simulink model "ASS_Final"  (R2019a)
settings: Solver=VariableStepAuto  StartTime=0.0  StopTime=30  RelTol=1e-3
values from neighbouring files (symbols this model uses):
  B1 = 100    [ASS_Final_parametros.m]
  B2 = 2000    [ASS_Final_parametros.m]
  eta = 0.92    [ASS_Final_parametros.m]
  io = 0    [ASS_Final_parametros.m]
  J = 0.15e-6    (= 1.5e-07)    [ASS_Final_parametros.m]
  k = 0.456    [ASS_Final_parametros.m]
  K1 = 125000    [ASS_Final_parametros.m]
  K2 = 28000    [ASS_Final_parametros.m]
  L = 20e-3    (= 0.02)    [ASS_Final_parametros.m]
  M1 = 40    [ASS_Final_parametros.m]
  M2 = 250    [ASS_Final_parametros.m]
  r = 0.4    [ASS_Final_parametros.m]
settings Model: Creator=luiso  LastModifiedBy=Amilcar A

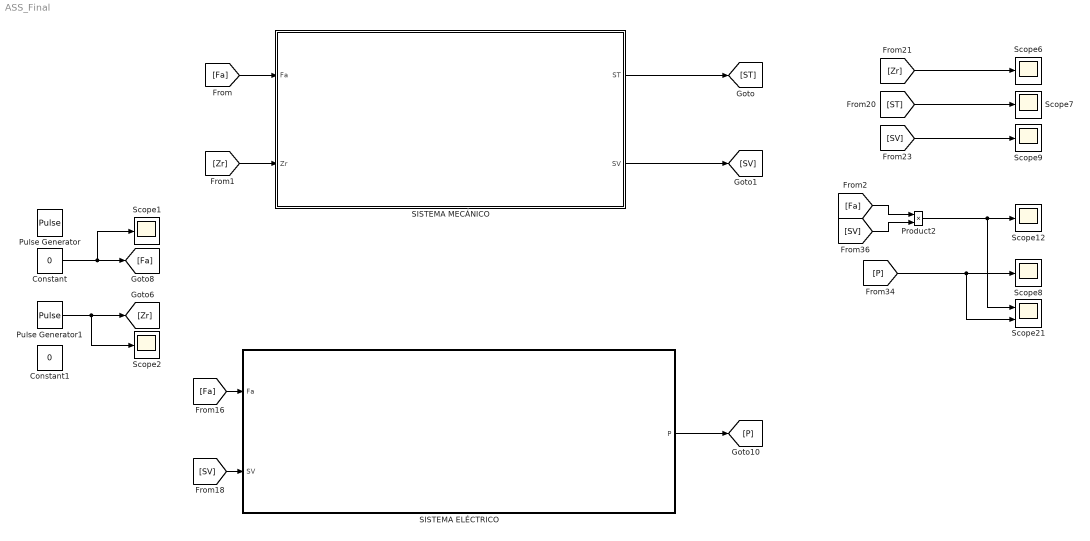
== system ASS_Final ==
  Constant : Constant  Value=0
  Constant1 : Constant  Value=0
  Product2 : Product
  Pulse Generator : DiscretePulseGenerator  PulseType=Time based  Amplitude=10  Period=10  PulseWidth=50
  Pulse Generator1 : DiscretePulseGenerator  PulseType=Time based  Amplitude=10e-4  Period=10  PulseWidth=50
  SISTEMA ELÉCTRICO : Subsystem
  SISTEMA MECÁNICO : Subsystem
  Scope{1..2,6..9,12} (7 alike) : Scope
  Scope21 : Scope  NumInputPorts=2
  wires:
  Pulse Generator1/1 -> Scope2/1, [Zr]
  Constant/1 -> Scope1/1, [Fa]
  [SV] -> Product2/2
  Product2/1 -> Scope21/1, Scope12/1
  [P] -> Scope21/2, Scope8/1
  [ST] -> Scope7/1
  [Zr] -> Scope6/1
  [SV] -> Scope9/1
  [Fa] -> SISTEMA MECÁNICO/1(Fa)
  [Zr] -> SISTEMA MECÁNICO/2(Zr)
  SISTEMA MECÁNICO/1(ST) -> [ST]
  SISTEMA MECÁNICO/2(SV) -> [SV]
  [Fa] -> SISTEMA ELÉCTRICO/1(Fa)
  [SV] -> SISTEMA ELÉCTRICO/2(SV)
  SISTEMA ELÉCTRICO/1(P) -> [P]
  [Fa] -> Product2/1

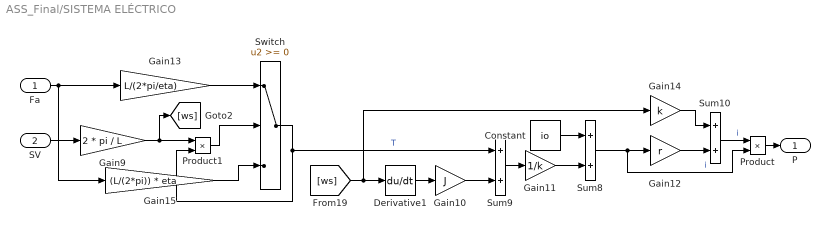
== system ASS_Final/SISTEMA ELÉCTRICO ==
  Fa : Inport
  SV : Inport  Port=2
  Constant : Constant  Value=io
  Derivative1 : Derivative
  Gain10 : Gain  Gain=J
  Gain11 : Gain  Gain=1/k
  Gain12 : Gain  Gain=r
  Gain13 : Gain  Gain=L/(2*pi/eta)
  Gain14 : Gain  Gain=k
  Gain15 : Gain  Gain=(L/(2*pi)) * eta
  Gain9 : Gain  Gain=2 * pi / L
  Product : Product
  Product1 : Product
  Sum10 : Sum
  Sum8 : Sum
  Sum9 : Sum
  Switch : Switch
  P : Outport
  wires:
  Constant/1 -> Sum8/1
  [ws] -> Gain14/1, Derivative1/1
  Gain15/1 -> Switch/3
  Switch/1 -> Product1/2, Sum9/1  "T"
  Gain12/1 -> Sum10/2
  Fa/1 -> Gain15/1, Gain13/1
  Sum9/1 -> Gain11/1
  Derivative1/1 -> Gain10/1
  Sum10/1 -> Product/1  "i"
  Gain10/1 -> Sum9/2
  Gain11/1 -> Sum8/2
  Product1/1 -> Switch/2
  Gain13/1 -> Switch/1
  Gain14/1 -> Sum10/1
  Product/1 -> P/1
  Sum8/1 -> Product/2, Gain12/1  "i"
  Gain9/1 -> [ws], Product1/1
  SV/1 -> Gain9/1

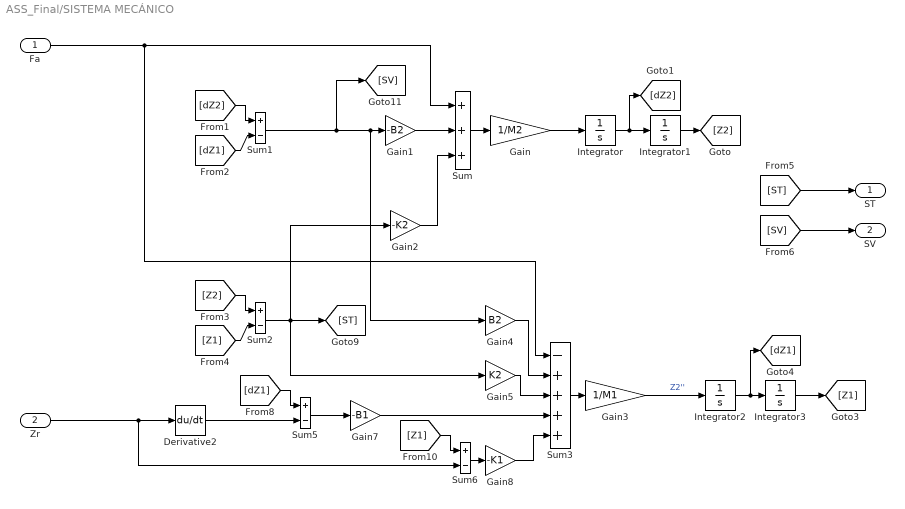
== system ASS_Final/SISTEMA MECÁNICO ==
  Fa : Inport
  Zr : Inport  Port=2
  Derivative2 : Derivative
  Gain : Gain  Gain=1/M2
  Gain1 : Gain  Gain=-B2
  Gain2 : Gain  Gain=-K2
  Gain3 : Gain  Gain=1/M1
  Gain4 : Gain  Gain=B2
  Gain5 : Gain  Gain=K2
  Gain7 : Gain  Gain=-B1
  Gain8 : Gain  Gain=-K1
  Integrator{,1..3} (4 alike) : Integrator
  Sum : Sum  Inputs=+++
  Sum{1..2,5..6} (4 alike) : Sum  Inputs=+-
  Sum3 : Sum  Inputs=-++++
  ST : Outport
  SV : Outport  Port=2
  wires:
  Gain/1 -> Integrator/1
  Sum1/1 -> Gain1/1, Gain4/1, [SV]
  Gain7/1 -> Sum3/4
  Sum2/1 -> Gain2/1, [ST], Gain5/1
  Gain8/1 -> Sum3/5
  Integrator3/1 -> [Z1]
  Sum6/1 -> Gain8/1
  Derivative2/1 -> Sum5/2
  Gain1/1 -> Sum/2
  Fa/1 -> Sum/1, Sum3/1
  Gain3/1 -> Integrator2/1  "Z2''"
  [Z1] -> Sum2/2
  Sum/1 -> Gain/1
  [Z2] -> Sum2/1
  Gain2/1 -> Sum/3
  [dZ1] -> Sum5/1
  Integrator/1 -> [dZ2], Integrator1/1
  [SV] -> SV/1
  Integrator1/1 -> [Z2]
  Gain4/1 -> Sum3/2
  Integrator2/1 -> [dZ1], Integrator3/1
  Sum5/1 -> Gain7/1
  Gain5/1 -> Sum3/3
  Sum3/1 -> Gain3/1
  [ST] -> ST/1
  [dZ2] -> Sum1/1
  Zr/1 -> Sum6/2, Derivative2/1
  [dZ1] -> Sum1/2
  [Z1] -> Sum6/1
